simulink model "model"  (R2023b)
settings: Solver=VariableStepAuto  StartTime=0.0  StopTime=1  RelTol=1e-3
undefined symbols (not defined in the file): A, b, d, g, L, M, R, y0
settings Model: Creator=cr  LastModifiedBy=cr

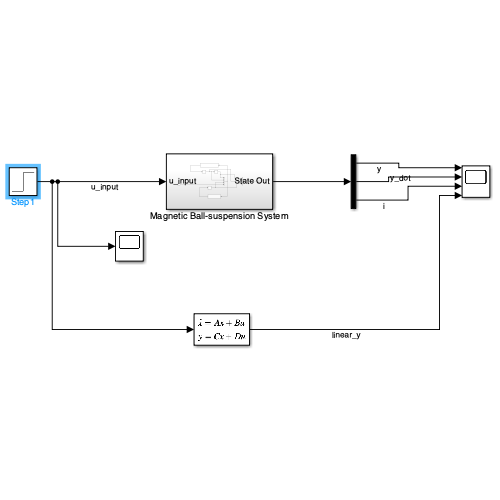
[thumbnail: Simulink's stored preview of the top-level diagram]
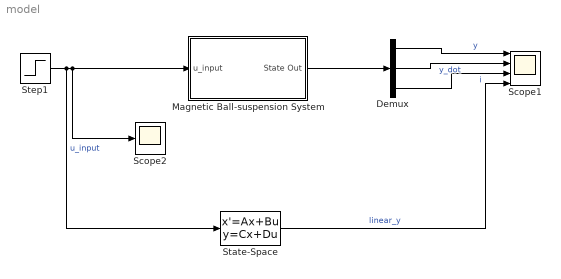
== system model ==
  Demux : Demux  Outputs=3
  Magnetic Ball-suspension System : Subsystem
  Scope1 : Scope  NumInputPorts=4
  Scope2 : Scope
  State-Space : StateSpace  A=A  B=b  C=c'  D=d  InitialCondition=[y0; 0; sqrt(M*g*y0^2)]
  Step1 : Step  Time=0.5  After=150  SampleTime=0
  wires:
  Step1/1 -> State-Space/1, Scope2/1, Magnetic Ball-suspension System/1(u_input)  "u_input"
  Magnetic Ball-suspension System/1(State Out) -> Demux/1
  Demux/2 -> Scope1/2  "y_dot"
  Demux/1 -> Scope1/1  "y"
  Demux/3 -> Scope1/3  "i"
  State-Space/1 -> Scope1/4  "linear_y"

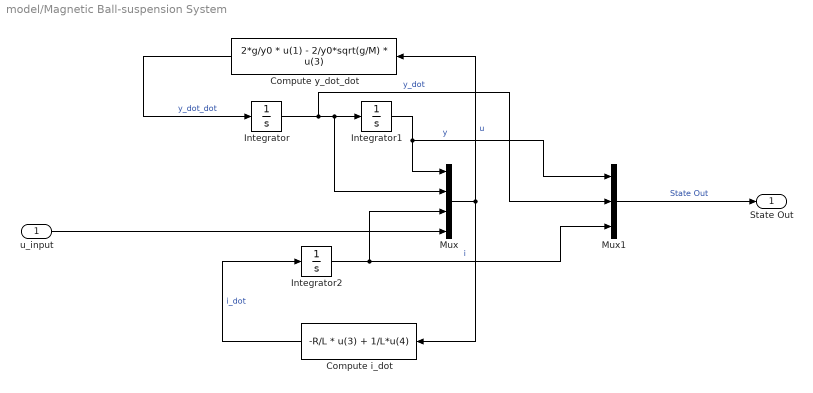
== system model/Magnetic Ball-suspension System ==
  u_input : Inport
  Compute i_dot : Fcn  Expr=-R/L * u(3) + 1/L*u(4)
  Compute y_dot_dot : Fcn  Expr=2*g/y0 * u(1) - 2/y0*sqrt(g/M) * u(3)
  Integrator : Integrator
  Integrator1 : Integrator  InitialCondition=y0
  Integrator2 : Integrator  InitialCondition=sqrt(M*g*y0^2)
  Mux : Mux
  Mux1 : Mux  Inputs=3
  State Out : Outport
  wires:
  Mux1/1 -> State Out/1  "State Out"
  Compute i_dot/1 -> Integrator2/1  "i_dot"
  Integrator/1 -> Mux1/2, Mux/2, Integrator1/1  "y_dot"
  Mux/1 -> Compute i_dot/1, Compute y_dot_dot/1  "u"
  Integrator2/1 -> Mux1/3, Mux/3  "i"
  u_input/1 -> Mux/4
  Compute y_dot_dot/1 -> Integrator/1  "y_dot_dot"
  Integrator1/1 -> Mux1/1, Mux/1  "y"
